simulink model "for_trim"  (R2020b)
settings: Solver=VariableStepAuto  StartTime=0.0  StopTime=10.0  RelTol=1e-3
values from neighbouring files (symbols this model uses):
  b = 9.144    [for_trimm.m]
  chord = 3.45    [for_trimm.m]
  d_SB = 0    [for_trimm.m]
  Mass = 9300    [for_trimm.m]
  S = 27.88    [for_trimm.m]
  X_cg = 0.35    [for_trimm.m]
  X_cg_ref = 0.35    [for_trimm.m]
undefined symbols (not defined in the file or in its folder): f16_database
libraries: simulink_extras x6, shared6dof x1, aerolibatmos2 x1, aerolibasang x1
(part 2 of 2)

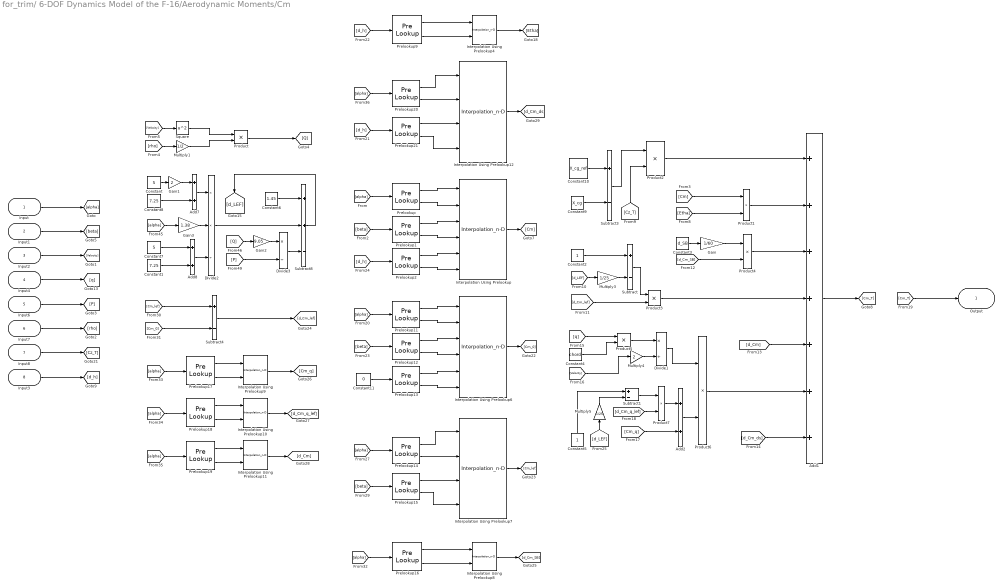
== system for_trim/ 6-DOF Dynamics Model of the F-16/Aerodynamic Moments/Cm ==
  Input : Inport
  Input1 : Inport  Port=2
  Input2 : Inport  Port=3
  Input4 : Inport  Port=4
  Input6 : Inport  Port=5
  Input7 : Inport  Port=6
  Input8 : Inport  Port=7
  Input3 : Inport  Port=8
  Add1 : Sum  Inputs=+++++++
  Add2 : Sum
  Add7 : Sum
  Add8 : Sum
  Constant : Constant  Value=S
  Constant1 : Constant  Value=7.25
  Constant10 : Constant  Value=X_cg_ref
  Constant11 : Constant  Value=0
  Constant2 : Constant
  Constant3 : Constant  Value=d_SB
  Constant4 : Constant  Value=chord
  Constant5 : Constant
  Constant6 : Constant  Value=1.45
  Constant7 : Constant  Value=S
  Constant8 : Constant  Value=7.25
  Constant9 : Constant  Value=X_cg
  Divide1 : Product  Inputs=*/
  Divide2 : Product  Inputs=**/
  Divide3 : Product  Inputs=*/
  Gain : Gain  Gain=1/60
  Gain1 : Gain  Gain=2
  Gain2 : Gain  Gain=9.05
  Gain3 : Gain  Gain=1.38
  Interpolation Using Prelookup : Interpolation_n-D  NumberOfTableDimensions=3  Table=f16_database.f16_AerodynamicData.data.Cm.Cm  InternalRulePriority=Speed
      settings: InputPortMap=u0,u1,u2,u3,u4,u5
  Interpolation Using Prelookup10 : Interpolation_n-D  NumberOfTableDimensions=1  Table=f16_database.f16_AerodynamicData.data.Cm.deltaCmqlef  InternalRulePriority=Speed
      settings: InputPortMap=u0,u1
  Interpolation Using Prelookup11 : Interpolation_n-D  NumberOfTableDimensions=1  Table=f16_database.f16_AerodynamicData.data.Cm.deltaCm  InternalRulePriority=Speed
      settings: InputPortMap=u0,u1
  Interpolation Using Prelookup12 : Interpolation_n-D  Table=f16_database.f16_AerodynamicData.data.Cm.deltaCmds  InternalRulePriority=Speed
  Interpolation Using Prelookup4 : Interpolation_n-D  NumberOfTableDimensions=1  Table=f16_database.f16_AerodynamicData.data.Cm.n_dHT  InternalRulePriority=Speed
      settings: InputPortMap=u0,u1
  Interpolation Using Prelookup6 : Interpolation_n-D  NumberOfTableDimensions=3  Table=f16_database.f16_AerodynamicData.data.Cm.Cm  InternalRulePriority=Speed
      settings: InputPortMap=u0,u1,u2,u3,u4,u5
  Interpolation Using Prelookup7 : Interpolation_n-D  Table=f16_database.f16_AerodynamicData.data.Cm.Cmlef  InternalRulePriority=Speed
  Interpolation Using Prelookup8 : Interpolation_n-D  NumberOfTableDimensions=1  Table=f16_database.f16_AerodynamicData.data.Cm.deltaCmSB  InternalRulePriority=Speed
      settings: InputPortMap=u0,u1
  Interpolation Using Prelookup9 : Interpolation_n-D  NumberOfTableDimensions=1  Table=f16_database.f16_AerodynamicData.data.Cm.Cmq  InternalRulePriority=Speed
      settings: InputPortMap=u0,u1
  Multiply1 : Gain  Gain=1/2
  Multiply3 : Gain  Gain=1/25
  Multiply4 : Gain  Gain=2
  Multiply5 : Gain  Gain=1/25
  Prelookup : PreLookup  BreakpointsData=f16_database.f16_AerodynamicData.BP.Cm.Cm.alpha  ExtrapMethod=Linear
  Prelookup1 : PreLookup  BreakpointsData=f16_database.f16_AerodynamicData.BP.Cm.Cm.beta  ExtrapMethod=Linear
  Prelookup11 : PreLookup  BreakpointsData=f16_database.f16_AerodynamicData.BP.Cm.Cm.alpha  ExtrapMethod=Linear
  Prelookup12 : PreLookup  BreakpointsData=f16_database.f16_AerodynamicData.BP.Cm.Cm.beta  ExtrapMethod=Linear
  Prelookup13 : PreLookup  BreakpointsData=f16_database.f16_AerodynamicData.BP.Cm.Cm.dHT  ExtrapMethod=Linear
  Prelookup14 : PreLookup  BreakpointsData=f16_database.f16_AerodynamicData.BP.Cm.Cmlef.alpha  ExtrapMethod=Linear
  Prelookup15 : PreLookup  BreakpointsData=f16_database.f16_AerodynamicData.BP.Cm.Cmlef.beta  ExtrapMethod=Linear
  Prelookup16 : PreLookup  BreakpointsData=f16_database.f16_AerodynamicData.BP.Cm.deltaCmSB.alpha  ExtrapMethod=Linear
  Prelookup17 : PreLookup  BreakpointsData=f16_database.f16_AerodynamicData.BP.Cm.Cmq.alpha  ExtrapMethod=Linear
  Prelookup18 : PreLookup  BreakpointsData=f16_database.f16_AerodynamicData.BP.Cm.deltaCmqlef.alpha  ExtrapMethod=Linear
  Prelookup19 : PreLookup  BreakpointsData=f16_database.f16_AerodynamicData.BP.Cm.deltaCm.alpha  ExtrapMethod=Linear
  Prelookup2 : PreLookup  BreakpointsData=f16_database.f16_AerodynamicData.BP.Cm.Cm.dHT  ExtrapMethod=Linear
  Prelookup20 : PreLookup  BreakpointsData=f16_database.f16_AerodynamicData.BP.Cm.deltaCmds.alpha  ExtrapMethod=Linear
  Prelookup21 : PreLookup  BreakpointsData=f16_database.f16_AerodynamicData.BP.Cm.deltaCmds.dHT  ExtrapMethod=Linear
  Prelookup9 : PreLookup  BreakpointsData=f16_database.f16_AerodynamicData.BP.Cm.n_dHT.dHT  ExtrapMethod=Linear
  Product{,1..7} (8 alike) : Product
  Square : Math  Operator=square  SaturateOnIntegerOverflow=on
  Subtract{,1,3..4} (4 alike) : Sum  Inputs=+-
  Subtract8 : Sum  Inputs=++-
  Output : Outport
  wires:
  Input1/1 -> [beta]
  Input2/1 -> [Velocity]
  Input4/1 -> [q]
  Input7/1 -> [rho]
  Input6/1 -> [P]
  Input/1 -> [alpha]
  Square/1 -> Product/1
  Interpolation Using Prelookup4/1 -> [Etha]
  Prelookup/2 -> Interpolation Using Prelookup/2
  Interpolation Using Prelookup/1 -> [Cm]
  Prelookup1/2 -> Interpolation Using Prelookup/4
  [rho] -> Multiply1/1
  Product/1 -> [Q]
  [beta] -> Prelookup1/1
  Multiply1/1 -> Product/2
  Prelookup1/1 -> Interpolation Using Prelookup/3
  [d_h] -> Prelookup2/1
  Prelookup2/1 -> Interpolation Using Prelookup/5
  Prelookup9/2 -> Interpolation Using Prelookup4/2
  Prelookup9/1 -> Interpolation Using Prelookup4/1
  [alpha] -> Prelookup/1
  Prelookup2/2 -> Interpolation Using Prelookup/6
  [Velocity] -> Square/1
  Prelookup/1 -> Interpolation Using Prelookup/1
  [d_h] -> Prelookup9/1
  Input8/1 -> [Cz_T]
  Constant10/1 -> Subtract3/1
  Constant9/1 -> Subtract3/2
  Prelookup11/1 -> Interpolation Using Prelookup6/1
  Prelookup13/2 -> Interpolation Using Prelookup6/6
  [alpha] -> Prelookup11/1
  Prelookup13/1 -> Interpolation Using Prelookup6/5
  Constant11/1 -> Prelookup13/1
  Prelookup12/1 -> Interpolation Using Prelookup6/3
  [beta] -> Prelookup12/1
  Prelookup12/2 -> Interpolation Using Prelookup6/4
  Interpolation Using Prelookup6/1 -> [Cm_0]
  Prelookup11/2 -> Interpolation Using Prelookup6/2
  Prelookup14/2 -> Interpolation Using Prelookup7/2
  Interpolation Using Prelookup7/1 -> [Cm_lef]
  Prelookup15/2 -> Interpolation Using Prelookup7/4
  [beta] -> Prelookup15/1
  Prelookup15/1 -> Interpolation Using Prelookup7/3
  [alpha] -> Prelookup14/1
  Prelookup14/1 -> Interpolation Using Prelookup7/1
  [Cm_lef] -> Subtract4/1
  [Cm_0] -> Subtract4/2
  Subtract4/1 -> [d_Cm_lef]
  Prelookup16/1 -> Interpolation Using Prelookup8/1
  Prelookup16/2 -> Interpolation Using Prelookup8/2
  Interpolation Using Prelookup8/1 -> [d_Cm_SB]
  [alpha] -> Prelookup16/1
  [alpha] -> Prelookup17/1
  Interpolation Using Prelookup9/1 -> [Cm_q]
  Prelookup17/2 -> Interpolation Using Prelookup9/2
  Prelookup17/1 -> Interpolation Using Prelookup9/1
  Prelookup18/1 -> Interpolation Using Prelookup10/1
  Prelookup18/2 -> Interpolation Using Prelookup10/2
  Interpolation Using Prelookup10/1 -> [d_Cm_q_lef]
  [alpha] -> Prelookup18/1
  [alpha] -> Prelookup19/1
  Interpolation Using Prelookup11/1 -> [d_Cm]
  Prelookup19/2 -> Interpolation Using Prelookup11/2
  Prelookup19/1 -> Interpolation Using Prelookup11/1
  Prelookup20/1 -> Interpolation Using Prelookup12/1
  [alpha] -> Prelookup20/1
  Prelookup21/1 -> Interpolation Using Prelookup12/3
  [d_h] -> Prelookup21/1
  Prelookup21/2 -> Interpolation Using Prelookup12/4
  Interpolation Using Prelookup12/1 -> [d_Cm_ds]
  Prelookup20/2 -> Interpolation Using Prelookup12/2
  [Cm] -> Product1/1
  [Etha] -> Product1/2
  Subtract3/1 -> Product2/1
  [Cz_T] -> Product2/2
  Constant2/1 -> Subtract/1
  [d_LEF] -> Multiply3/1
  Multiply3/1 -> Subtract/2
  Subtract/1 -> Product3/1
  [d_Cm_lef] -> Product3/2
  [d_Cm_SB] -> Product4/2
  Gain/1 -> Product4/1
  Constant3/1 -> Gain/1
  Product7/1 -> Add2/1
  [Cm_q] -> Add2/2
  Divide1/1 -> Product6/1
  Product6/1 -> Add1/6
  Multiply5/1 -> Subtract1/2
  [d_Cm_q_lef] -> Product7/2
  Multiply4/1 -> Divide1/2
  [Velocity] -> Multiply4/1
  [q] -> Product5/1
  Add2/1 -> Product6/2
  Product5/1 -> Divide1/1
  [d_LEF] -> Multiply5/1
  Subtract1/1 -> Product7/1
  Constant5/1 -> Subtract1/1
  Constant4/1 -> Product5/2
  [d_Cm_ds] -> Add1/7
  [d_Cm] -> Add1/5
  Product3/1 -> Add1/4
  Product2/1 -> Add1/1
  Product4/1 -> Add1/3
  Product1/1 -> Add1/2
  Add1/1 -> [Cm_T]
  [Cm_T] -> Output/1
  Input3/1 -> [d_h]
  Add8/1 -> Divide2/3
  Add7/1 -> Divide2/1
  Divide3/1 -> Subtract8/3
  [alpha] -> Gain3/1
  Gain2/1 -> Divide3/1
  Subtract8/1 -> [d_LEF]
  Constant1/1 -> Add8/2
  Divide2/1 -> Subtract8/2
  Constant7/1 -> Add8/1
  Gain1/1 -> Add7/1
  [Q] -> Gain2/1
  Constant6/1 -> Subtract8/1
  Constant/1 -> Gain1/1
  [P] -> Divide3/2
  Gain3/1 -> Divide2/2
  Constant8/1 -> Add7/2

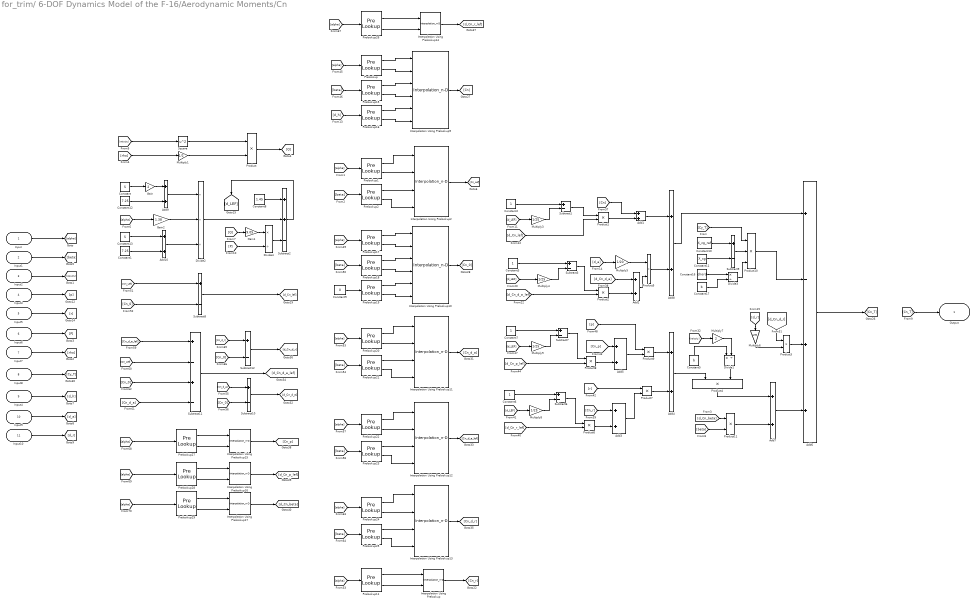
== system for_trim/ 6-DOF Dynamics Model of the F-16/Aerodynamic Moments/Cn ==
  Input : Inport
  Input1 : Inport  Port=2
  Input2 : Inport  Port=3
  Input3 : Inport  Port=4
  Input5 : Inport  Port=5
  Input6 : Inport  Port=6
  Input7 : Inport  Port=7
  Input8 : Inport  Port=8
  Input4 : Inport  Port=9
  Input9 : Inport  Port=10
  Input10 : Inport  Port=11
  Add{1..5,7..10} (9 alike) : Sum
  Add6 : Sum  Inputs=+-++
  Constant : Constant  Value=S
  Constant1 : Constant  Value=7.25
  Constant10 : Constant  Value=X_cg_ref
  Constant11 : Constant  Value=X_cg
  Constant12 : Constant  Value=7.25
  Constant13 : Constant  Value=S
  Constant16 : Constant  Value=chord
  Constant17 : Constant  Value=b
  Constant{2..3,6..7} (4 alike) : Constant
  Constant5 : Constant  Value=b
  Constant8 : Constant  Value=1.45
  Constant9 : Constant  Value=0
  Divide1 : Product  Inputs=*/
  Divide2 : Product  Inputs=**/
  Divide3 : Product  Inputs=*/
  Divide4 : Product  Inputs=*/
  Gain : Gain  Gain=2
  Gain1 : Gain  Gain=9.05
  Gain2 : Gain  Gain=1.38
  Interpolation Using Prelookup : Interpolation_n-D  NumberOfTableDimensions=1  Table=f16_database.f16_AerodynamicData.data.Cn.Cnr  InternalRulePriority=Speed
      settings: InputPortMap=u0,u1
  Interpolation Using Prelookup10 : Interpolation_n-D  NumberOfTableDimensions=3  Table=f16_database.f16_AerodynamicData.data.Cn.Cn  InternalRulePriority=Speed
      settings: InputPortMap=u0,u1,u2,u3,u4,u5
  Interpolation Using Prelookup11 : Interpolation_n-D  Table=f16_database.f16_AerodynamicData.data.Cn.Cnda20  InternalRulePriority=Speed
  Interpolation Using Prelookup12 : Interpolation_n-D  Table=f16_database.f16_AerodynamicData.data.Cn.Cnda20lef  InternalRulePriority=Speed
  Interpolation Using Prelookup13 : Interpolation_n-D  Table=f16_database.f16_AerodynamicData.data.Cn.Cndr30  InternalRulePriority=Speed
  Interpolation Using Prelookup14 : Interpolation_n-D  NumberOfTableDimensions=1  Table=f16_database.f16_AerodynamicData.data.Cn.deltaCnrlef  InternalRulePriority=Speed
      settings: InputPortMap=u0,u1
  Interpolation Using Prelookup15 : Interpolation_n-D  NumberOfTableDimensions=1  Table=f16_database.f16_AerodynamicData.data.Cn.Cnp  InternalRulePriority=Speed
      settings: InputPortMap=u0,u1
  Interpolation Using Prelookup16 : Interpolation_n-D  NumberOfTableDimensions=1  Table=f16_database.f16_AerodynamicData.data.Cn.deltaCnplef  InternalRulePriority=Speed
      settings: InputPortMap=u0,u1
  Interpolation Using Prelookup17 : Interpolation_n-D  NumberOfTableDimensions=1  Table=f16_database.f16_AerodynamicData.data.Cn.deltaCnBeta  InternalRulePriority=Speed
      settings: InputPortMap=u0,u1
  Interpolation Using Prelookup2 : Interpolation_n-D  Table=f16_database.f16_AerodynamicData.data.Cn.Cnlef  InternalRulePriority=Speed
  Interpolation Using Prelookup9 : Interpolation_n-D  NumberOfTableDimensions=3  Table=f16_database.f16_AerodynamicData.data.Cn.Cn  InternalRulePriority=Speed
      settings: InputPortMap=u0,u1,u2,u3,u4,u5
  Multiply1 : Gain  Gain=1/2
  Multiply{3..4,8..9} (4 alike) : Gain  Gain=1/25
  Multiply5 : Gain  Gain=1/20
  Multiply6 : Gain  Gain=1/30
  Multiply7 : Gain  Gain=2
  Prelookup : PreLookup  BreakpointsData=f16_database.f16_AerodynamicData.BP.Cn.Cn.alpha  ExtrapMethod=Linear
  Prelookup1 : PreLookup  BreakpointsData=f16_database.f16_AerodynamicData.BP.Cn.Cnlef.alpha  ExtrapMethod=Linear
  Prelookup11 : PreLookup  BreakpointsData=f16_database.f16_AerodynamicData.BP.Cn.Cnr.alpha  ExtrapMethod=Linear
  Prelookup15 : PreLookup  BreakpointsData=f16_database.f16_AerodynamicData.BP.Cn.Cn.beta  ExtrapMethod=Linear
  Prelookup16 : PreLookup  BreakpointsData=f16_database.f16_AerodynamicData.BP.Cn.Cn.dHT  ExtrapMethod=Linear
  Prelookup17 : PreLookup  BreakpointsData=f16_database.f16_AerodynamicData.BP.Cn.Cn.alpha  ExtrapMethod=Linear
  Prelookup18 : PreLookup  BreakpointsData=f16_database.f16_AerodynamicData.BP.Cn.Cn.beta  ExtrapMethod=Linear
  Prelookup19 : PreLookup  BreakpointsData=f16_database.f16_AerodynamicData.BP.Cn.Cn.dHT  ExtrapMethod=Linear
  Prelookup2 : PreLookup  BreakpointsData=f16_database.f16_AerodynamicData.BP.Cn.Cnlef.beta  ExtrapMethod=Linear
  Prelookup20 : PreLookup  BreakpointsData=f16_database.f16_AerodynamicData.BP.Cn.Cnda20.alpha  ExtrapMethod=Linear
  Prelookup21 : PreLookup  BreakpointsData=f16_database.f16_AerodynamicData.BP.Cn.Cnda20.beta  ExtrapMethod=Linear
  Prelookup22 : PreLookup  BreakpointsData=f16_database.f16_AerodynamicData.BP.Cn.Cnda20lef.alpha  ExtrapMethod=Linear
  Prelookup23 : PreLookup  BreakpointsData=f16_database.f16_AerodynamicData.BP.Cn.Cnda20lef.beta  ExtrapMethod=Linear
  Prelookup24 : PreLookup  BreakpointsData=f16_database.f16_AerodynamicData.BP.Cn.Cndr30.alpha  ExtrapMethod=Linear
  Prelookup25 : PreLookup  BreakpointsData=f16_database.f16_AerodynamicData.BP.Cn.Cndr30.beta  ExtrapMethod=Linear
  Prelookup26 : PreLookup  BreakpointsData=f16_database.f16_AerodynamicData.BP.Cn.deltaCnrlef.alpha  ExtrapMethod=Linear
  Prelookup27 : PreLookup  BreakpointsData=f16_database.f16_AerodynamicData.BP.Cn.Cnp.alpha  ExtrapMethod=Linear
  Prelookup28 : PreLookup  BreakpointsData=f16_database.f16_AerodynamicData.BP.Cn.deltaCnplef.alpha  ExtrapMethod=Linear
  Prelookup29 : PreLookup  BreakpointsData=f16_database.f16_AerodynamicData.BP.Cn.deltaCnBeta.alpha  ExtrapMethod=Linear
  Product{,1..9,11} (11 alike) : Product
  Product10 : Product  Inputs=3
  Square : Math  Operator=square  SaturateOnIntegerOverflow=on
  Subtract{1,3,6..10,12} (8 alike) : Sum  Inputs=+-
  Subtract11 : Sum  Inputs=+-+-
  Subtract2 : Sum  Inputs=++-
  Output : Outport
  wires:
  Add6/1 -> [Cn_T]
  Add4/1 -> Product4/1
  Divide1/1 -> Product4/2
  Product9/1 -> Add4/1
  Constant7/1 -> Subtract7/1
  [d_LEF] -> Multiply9/1
  Subtract7/1 -> Product8/1
  Multiply9/1 -> Subtract7/2
  [d_Cn_p_lef] -> Product8/2
  [Cn_p] -> Add5/1
  Product8/1 -> Add5/2
  Add5/1 -> Product9/2
  [p] -> Product9/1
  Product7/1 -> Add4/2
  [r] -> Product7/1
  Add3/1 -> Product7/2
  Product6/1 -> Add3/2
  [Cn_r] -> Add3/1
  [d_Cn_r_lef] -> Product6/2
  Multiply8/1 -> Subtract6/2
  Subtract6/1 -> Product6/1
  [d_LEF] -> Multiply8/1
  Constant6/1 -> Subtract6/1
  Multiply5/1 -> Product5/1
  Add2/1 -> Product5/2
  [d_Cn_d_a] -> Add2/1
  Product1/1 -> Add1/2
  [Cn] -> Add1/1
  Interpolation Using Prelookup/1 -> [Cn_r]
  Prelookup11/2 -> Interpolation Using Prelookup/2
  Prelookup11/1 -> Interpolation Using Prelookup/1
  [alpha] -> Prelookup11/1
  Multiply7/1 -> Divide1/2
  [Velocity] -> Multiply7/1
  Constant5/1 -> Divide1/1
  [d_r] -> Multiply6/1
  [d_a] -> Multiply5/1
  Constant3/1 -> Subtract3/1
  [d_Cn_d_a_lef] -> Product2/2
  Product2/1 -> Add2/2
  Multiply4/1 -> Subtract3/2
  [d_LEF] -> Multiply4/1
  Subtract3/1 -> Product2/1
  Subtract1/1 -> Product1/1
  Multiply3/1 -> Subtract1/2
  Constant2/1 -> Subtract1/1
  [d_Cn_lef] -> Product1/2
  [d_LEF] -> Multiply3/1
  Interpolation Using Prelookup2/1 -> [Cn_Lef]
  Prelookup2/1 -> Interpolation Using Prelookup2/3
  [beta] -> Prelookup2/1
  Prelookup1/1 -> Interpolation Using Prelookup2/1
  Prelookup2/2 -> Interpolation Using Prelookup2/4
  [alpha] -> Prelookup1/1
  Prelookup1/2 -> Interpolation Using Prelookup2/2
  [Cn_T] -> Output/1
  Input1/1 -> [beta]
  Input2/1 -> [Velocity]
  Input7/1 -> [rho]
  Input6/1 -> [P]
  Input5/1 -> [r]
  Input3/1 -> [p]
  Input/1 -> [alpha]
  Square/1 -> Product/1
  [rho] -> Multiply1/1
  Product/1 -> [Q]
  Multiply1/1 -> Product/2
  [Velocity] -> Square/1
  Interpolation Using Prelookup9/1 -> [Cn]
  Prelookup15/2 -> Interpolation Using Prelookup9/4
  Prelookup15/1 -> Interpolation Using Prelookup9/3
  Prelookup16/2 -> Interpolation Using Prelookup9/6
  [d_h] -> Prelookup16/1
  Prelookup/1 -> Interpolation Using Prelookup9/1
  Prelookup16/1 -> Interpolation Using Prelookup9/5
  Prelookup/2 -> Interpolation Using Prelookup9/2
  [alpha] -> Prelookup/1
  [beta] -> Prelookup15/1
  [beta] -> Prelookup18/1
  [alpha] -> Prelookup17/1
  Prelookup17/2 -> Interpolation Using Prelookup10/2
  Prelookup19/1 -> Interpolation Using Prelookup10/5
  Prelookup17/1 -> Interpolation Using Prelookup10/1
  Constant9/1 -> Prelookup19/1
  Prelookup19/2 -> Interpolation Using Prelookup10/6
  Prelookup18/1 -> Interpolation Using Prelookup10/3
  Prelookup18/2 -> Interpolation Using Prelookup10/4
  Interpolation Using Prelookup10/1 -> [Cn_0]
  [Cn_Lef] -> Subtract8/1
  [Cn_0] -> Subtract8/2
  Subtract8/1 -> [d_Cn_lef]
  Input8/1 -> [Cy_T]
  Prelookup20/2 -> Interpolation Using Prelookup11/2
  [alpha] -> Prelookup20/1
  Prelookup21/2 -> Interpolation Using Prelookup11/4
  Prelookup20/1 -> Interpolation Using Prelookup11/1
  [beta] -> Prelookup21/1
  Prelookup21/1 -> Interpolation Using Prelookup11/3
  Interpolation Using Prelookup11/1 -> [Cn_d_a]
  Subtract10/1 -> [d_Cn_d_a]
  [Cn_0] -> Subtract10/2
  [Cn_d_a] -> Subtract10/1
  Interpolation Using Prelookup12/1 -> [Cn_d_a_lef]
  Prelookup23/1 -> Interpolation Using Prelookup12/3
  [beta] -> Prelookup23/1
  Prelookup22/1 -> Interpolation Using Prelookup12/1
  Prelookup23/2 -> Interpolation Using Prelookup12/4
  [alpha] -> Prelookup22/1
  Prelookup22/2 -> Interpolation Using Prelookup12/2
  [Cn_d_a_lef] -> Subtract11/1
  [Cn_Lef] -> Subtract11/2
  [Cn_d_a] -> Subtract11/4
  [Cn_0] -> Subtract11/3
  Subtract11/1 -> [d_Cn_d_a_lef]
  Prelookup24/2 -> Interpolation Using Prelookup13/2
  [alpha] -> Prelookup24/1
  Prelookup25/2 -> Interpolation Using Prelookup13/4
  Prelookup24/1 -> Interpolation Using Prelookup13/1
  [beta] -> Prelookup25/1
  Prelookup25/1 -> Interpolation Using Prelookup13/3
  Interpolation Using Prelookup13/1 -> [Cn_d_r]
  [Cn_d_r] -> Subtract12/1
  [Cn_0] -> Subtract12/2
  Subtract12/1 -> [d_Cn_d_r]
  [alpha] -> Prelookup26/1
  Prelookup26/1 -> Interpolation Using Prelookup14/1
  Prelookup26/2 -> Interpolation Using Prelookup14/2
  Interpolation Using Prelookup14/1 -> [d_Cn_r_lef]
  Interpolation Using Prelookup15/1 -> [Cn_p]
  Prelookup27/2 -> Interpolation Using Prelookup15/2
  Prelookup27/1 -> Interpolation Using Prelookup15/1
  [alpha] -> Prelookup27/1
  [alpha] -> Prelookup28/1
  Prelookup28/1 -> Interpolation Using Prelookup16/1
  Prelookup28/2 -> Interpolation Using Prelookup16/2
  Interpolation Using Prelookup16/1 -> [d_Cn_p_lef]
  Interpolation Using Prelookup17/1 -> [d_Cn_beta]
  Prelookup29/2 -> Interpolation Using Prelookup17/2
  Prelookup29/1 -> Interpolation Using Prelookup17/1
  [alpha] -> Prelookup29/1
  Constant10/1 -> Subtract9/1
  Constant11/1 -> Subtract9/2
  Subtract9/1 -> Product10/2
  [Cy_T] -> Product10/1
  Constant16/1 -> Divide3/1
  Constant17/1 -> Divide3/2
  Divide3/1 -> Product10/3
  [d_Cn_beta] -> Product11/1
  [beta] -> Product11/2
  Product4/1 -> Add7/1
  Product11/1 -> Add7/2
  Add7/1 -> Add6/4
  Multiply6/1 -> Product3/2
  [d_Cn_d_r] -> Product3/1
  Product3/1 -> Add6/3
  Add1/1 -> Add8/1
  Product5/1 -> Add8/2
  Product10/1 -> Add6/2
  Add8/1 -> Add6/1
  Input4/1 -> [d_h]
  Input9/1 -> [d_a]
  Add10/1 -> Divide2/3
  Add9/1 -> Divide2/1
  Divide4/1 -> Subtract2/3
  [alpha] -> Gain2/1
  Gain1/1 -> Divide4/1
  Subtract2/1 -> [d_LEF]
  Constant1/1 -> Add10/2
  Divide2/1 -> Subtract2/2
  Constant13/1 -> Add10/1
  Gain/1 -> Add9/1
  [Q] -> Gain1/1
  Constant8/1 -> Subtract2/1
  Constant/1 -> Gain/1
  [P] -> Divide4/2
  Gain2/1 -> Divide2/2
  Constant12/1 -> Add9/2
  Input10/1 -> [d_r]

== system for_trim/ 6-DOF Dynamics Model of the F-16/Thrust/If Action Subsystem ==
  In1 : Inport
  Action Port : ActionPort  ActionPortLabel=if(u1< 50)
  Out1 : Outport
  wires:
  In1/1 -> Out1/1

== system for_trim/ 6-DOF Dynamics Model of the F-16/Thrust/If Action Subsystem1 ==
  In1 : Inport
  Action Port : ActionPort  ActionPortLabel=else
  Out1 : Outport
  wires:
  In1/1 -> Out1/1
